simulink model "Porownanie"  (R2017a)
settings: Solver=VariableStepAuto  StartTime=0.0  StopTime=200  RelTol=1e-3
values from neighbouring files (symbols this model uses):
  A = pi*R1*R1    (= 10.9999393421)    [Lab2.m]    (also in ModelDataNonlinear.m)
  B = (pi*R2*R2)/(3*H2*H2)    (= 0.00337009933323)    [Lab2.m]    (also in Lab8.m = deltah20max / k; Lab9.m = 0.4; ModelDataNonlinear.m)
  C1 = 1.372    [Lab2.m]    (also in ModelDataNonlinear.m)
  C2 = 0.332756    [Lab2.m]    (also in ModelDataNonlinear.m)
  deltaq1 = 0.1*q10    [Lab2.m]
  h10 = (q10/C1).^2    [Lab2.m]    (also in ModelDataNonlinear.m)
  h20 = h2max/2    (= 8)    [Lab2.m]    (also in ModelDataNonlinear.m)
  k = 5    [Lab1.m]    (also in Lab2.m = (2*sqrt(h20))/C2; ModelData.m = 17)
  q10 = C2*sqrt(h20)    [Lab2.m]    (also in ModelDataNonlinear.m)
  T1 = 3    [Lab1.m]    (also in Lab2.m = 2*pi*R1*R1*sqrt(h10)/C1; ModelData.m = 10.998)
  T2 = 4    [Lab1.m]    (also in Lab2.m = 2*A*sqrt(h10)/C1; ModelData.m = 10.998)
settings Model: Creator=ishiguro  LastModifiedBy=ishiguro

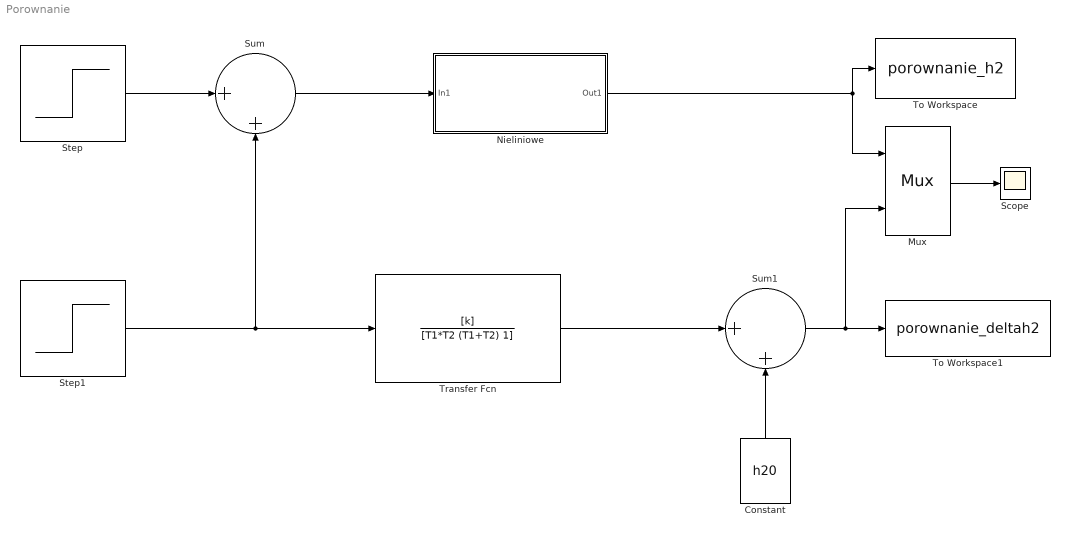
== system Porownanie ==
  Constant : Constant  Value=h20
  Mux : Mux  Inputs=2
      settings: DisplayOption=signals
  "Nieliniowe " : Subsystem
  Scope : Scope
  Step : Step  Time=0  After=q10  SampleTime=0
  Step1 : Step  Time=0  After=deltaq1  SampleTime=0
  Sum : Sum  Inputs=|++
  Sum1 : Sum  Inputs=|++
  To Workspace : ToWorkspace  VariableName=porownanie_h2  SampleTime=-1
  To Workspace1 : ToWorkspace  VariableName=porownanie_deltah2  SampleTime=-1
  Transfer Fcn : TransferFcn  Numerator=[k]  Denominator=[T1*T2 (T1+T2) 1]
  wires:
  Mux/1 -> Scope/1
  Sum/1 -> "Nieliniowe "/1(In1)
  Step/1 -> Sum/1
  Step1/1 -> Sum/2, Transfer Fcn/1
  Transfer Fcn/1 -> Sum1/1
  Constant/1 -> Sum1/2
  Sum1/1 -> To Workspace1/1, Mux/2
  "Nieliniowe "/1(Out1) -> Mux/1, To Workspace/1

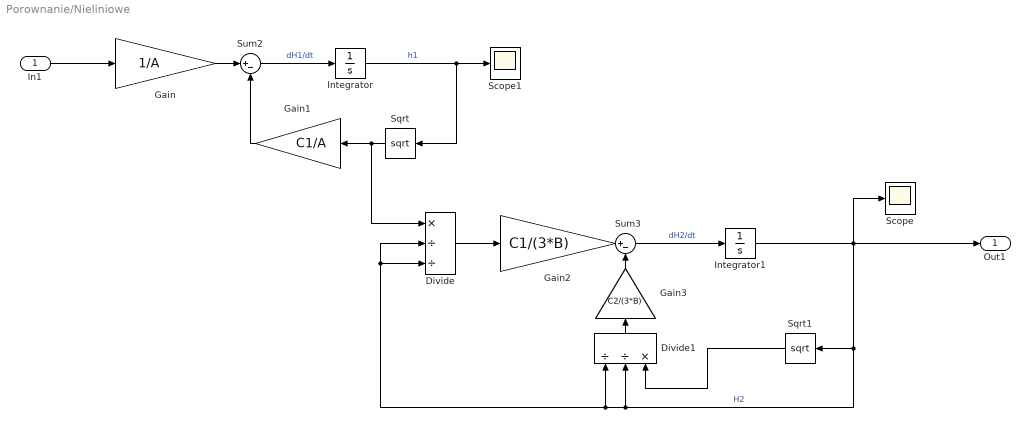
== system Porownanie/Nieliniowe  ==
  In1 : Inport
  Divide : Product  Inputs=*//
  Divide1 : Product  Inputs=//*
  Gain : Gain  Gain=1/A
  Gain1 : Gain  Gain=C1/A
  Gain2 : Gain  Gain=C1/(3*B)
  Gain3 : Gain  Gain=C2/(3*B)
  Integrator : Integrator  InitialCondition=h10
  Integrator1 : Integrator  InitialCondition=h20
  Scope : Scope
  Scope1 : Scope
  Sqrt : Sqrt  SaturateOnIntegerOverflow=on
  Sqrt1 : Sqrt  SaturateOnIntegerOverflow=on
  Sum2 : Sum  Inputs=|+-
  Sum3 : Sum  Inputs=|+-
  Out1 : Outport
  wires:
  Gain1/1 -> Sum2/2
  Gain/1 -> Sum2/1
  Sum2/1 -> Integrator/1  "dH1/dt"
  Integrator/1 -> Sqrt/1, Scope1/1  "h1"
  Integrator1/1 -> Scope/1, Out1/1, Sqrt1/1, Divide1/2, Divide1/1, Divide/3, Divide/2  "H2"
  Sum3/1 -> Integrator1/1  "dH2/dt"
  In1/1 -> Gain/1
  Divide/1 -> Gain2/1
  Gain2/1 -> Sum3/1
  Sqrt/1 -> Gain1/1, Divide/1
  Gain3/1 -> Sum3/2
  Divide1/1 -> Gain3/1
  Sqrt1/1 -> Divide1/3
